simulink model "task3_simulink_model"  (R2022b)
settings: Solver=FixedStepAuto  StartTime=0.0  StopTime=2  FixedStep=0.000001  RelTol=1e-3
undefined symbols (not defined in the file or in its folder): J, K_d, K_i, K_p, L_a, M_nom, Psi_nom, R_a, T_delta, U_nom
settings Model: Creator=Family  LastModifiedBy=R1300-W-5-Stud
settings ModelReferenceCC: EnableRefExpFcnMdlSchedulingChecks=on

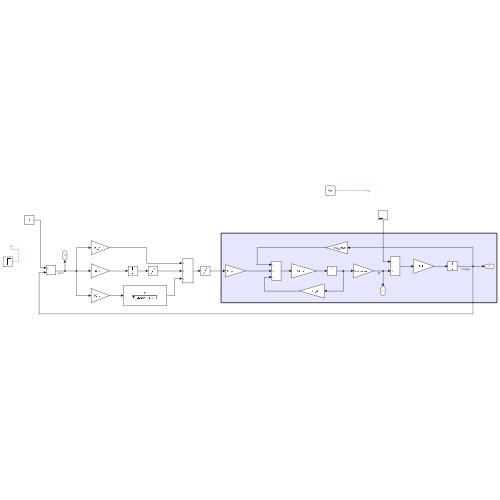
[thumbnail: Simulink's stored preview of the top-level diagram]
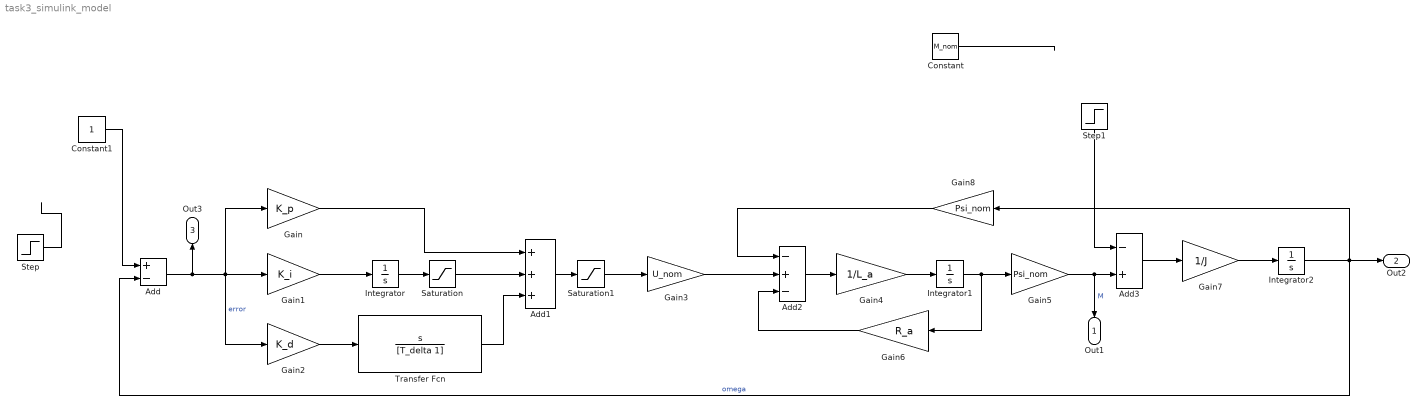
== system task3_simulink_model ==
  Add : Sum  Inputs=+-
  Add1 : Sum  Inputs=+++
  Add2 : Sum  Inputs=-+-
  Add3 : Sum  Inputs=-+
  Constant : Constant  Value=M_nom
  Constant1 : Constant
  Gain : Gain  Gain=K_p
  Gain1 : Gain  Gain=K_i
  Gain2 : Gain  Gain=K_d
  Gain3 : Gain  Gain=U_nom
  Gain4 : Gain  Gain=1/L_a
  Gain5 : Gain  Gain=Psi_nom
  Gain6 : Gain  Gain=R_a
  Gain7 : Gain  Gain=1/J
  Gain8 : Gain  Gain=Psi_nom
  Integrator : Integrator
  Integrator1 : Integrator
  Integrator2 : Integrator
  Saturation : Saturate  UpperLimit=1  LowerLimit=-1
  Saturation1 : Saturate  UpperLimit=1  LowerLimit=-1
  Step : Step  SampleTime=0.00001
  Step1 : Step  Before=0.5 * M_nom  After=M_nom  SampleTime=0
  Transfer Fcn : TransferFcn  Numerator=[1 0]  Denominator=[T_delta 1]
  Out1 : Outport
  Out2 : Outport  Port=2
  Out3 : Outport  Port=3
  wires:
  Gain/1 -> Add1/1
  Gain1/1 -> Integrator/1
  Gain2/1 -> Transfer Fcn/1
  Integrator/1 -> Saturation/1
  Saturation/1 -> Add1/2
  Add1/1 -> Saturation1/1
  Transfer Fcn/1 -> Add1/3
  Add/1 -> Out3/1, Gain/1, Gain2/1, Gain1/1  "error"
  Add3/1 -> Gain7/1
  Integrator2/1 -> Gain8/1, Add/2, Out2/1  "omega"
  Gain7/1 -> Integrator2/1
  Step1/1 -> Add3/1
  Gain6/1 -> Add2/3
  Gain5/1 -> Add3/2, Out1/1  "M"
  Gain4/1 -> Integrator1/1
  Add2/1 -> Gain4/1
  Gain3/1 -> Add2/2
  Integrator1/1 -> Gain6/1, Gain5/1
  Gain8/1 -> Add2/1
  Saturation1/1 -> Gain3/1
  Constant1/1 -> Add/1
  Step/1 -> ?
  Constant/1 -> ?
